simulink model "TappedDelay"  (R2017b)
settings: Solver=FixedStepDiscrete  StartTime=0.0  StopTime=20  FixedStep=1.000000  RelTol=1e-3
libraries: simulink x2
settings Model: Creator=hbourbou  LastModifiedBy=hbourbou
settings OptimizationCC: LifeSpan=inf
settings DebuggingCC: SFExecutionAtInitializationDiag=none
settings HardwareCC: ProdBitPerSizeT=32  ProdBitPerPtrDiffT=32  ProdWordSize=32  ProdHWDeviceType=Specified
settings CodeAppCC: StateflowObjectComments=on

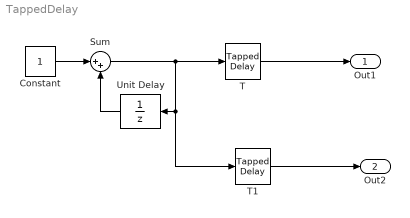
== system TappedDelay ==
  Constant : Constant  SampleTime=1
  Sum : Sum  Inputs=|++
  T : simulink/Discrete/Tapped Delay  vinit=0.0  samptime=-1  NumDelays=4  DelayOrder=Oldest  includeCurrent=off
  T1 : simulink/Discrete/Tapped Delay  vinit=0.0  samptime=-1  NumDelays=4  DelayOrder=Newest  includeCurrent=on
  Unit Delay : UnitDelay
  Out1 : Outport
  Out2 : Outport  Port=2
  wires:
  T/1 -> Out1/1
  Constant/1 -> Sum/1
  Sum/1 -> T/1, T1/1, Unit Delay/1
  Unit Delay/1 -> Sum/2
  T1/1 -> Out2/1
